simulink model "c_slow_test_cases"  (R2017a)
settings: Solver=FixedStepDiscrete  StartTime=0  StopTime=1000/5e6  RelTol=1e-3
libraries: helperLib x2, simulink x2, commrandsrc3 x2, dspsrcs4 x2
settings Model: FPTRunName=FPA_Reference  SimulationMode=accelerator  ExtModeTrigDuration=100  Creator=cyarp  LastModifiedBy=cyarp
settings SolverCC: InsertRTBMode=Always
settings DataIOCC: LimitDataPoints=on  SaveFinalState=on  SaveFormat=StructureWithTime  SaveOutput=off  SaveState=on  StateSaveName=tmp_raccel_xout  SignalLoggingName=tmp_raccel_logsout
settings OptimizationCC: BlockReduction=off  ConditionallyExecuteInputs=off  DefaultParameterBehavior=Inlined  EfficientMapNaN2IntZero=off  LifeSpan=inf  SimCompilerOptimization=on
settings DebuggingCC: AlgebraicLoopMsg=error  SolverPrmCheckMsg=warning  SingleTaskRateTransMsg=error  SFUnexpectedBacktrackingDiag=warning  SFNoUnconditionalDefaultTransitionDiag=warning  SFExecutionAtInitializationDiag=none
settings HardwareCC: ProdBitPerPointer=32  ProdBitPerSizeT=32  ProdBitPerPtrDiffT=32  ProdLargestAtomicFloat=None  ProdIntDivRoundTo=Undefined  ProdEndianess=Unspecified  ProdWordSize=32  ProdHWDeviceType=ASIC/FPGA->ASIC/FPGA  TargetBitPerPointer=64  TargetBitPerSizeT=64  TargetBitPerPtrDiffT=64  TargetLongLongMode=on  TargetIntDivRoundTo=Zero  TargetEndianess=LittleEndian  TargetWordSize=64  TargetHWDeviceType=MATLAB Host  ProdEqTarget=off
settings ModelReferenceCC: PropagateSignalLabelsOutOfModel=off
settings RTWCC: SystemTargetFile=raccel.tlc  TemplateMakefile=raccel_default_tmf  RTWVerbose=off  RTWUseSimCustomCode=on
settings CodeAppCC: GenerateComments=off  MaxIdLength=128  SimulinkBlockComments=off
settings RaccelTargetCC: GeneratePreprocessorConditionals=Use local settings  ERTFirstTimeCompliant=off  MultiInstanceERTCode=off  ExtModeMexArgs='', 0, 55180  ENABLE_SLEXEC_SSBRIDGE=11  RTWCAPISignals=off  RTWCAPIParams=on
settings ConfigComp: CovMetricSettings=dw  CovHtmlReporting=on  CovSaveCumulativeToWorkspaceVar=on  CovSaveSingleToWorkspaceVar=on  CovExternalEMLEnable=off  CovSFcnEnable=off

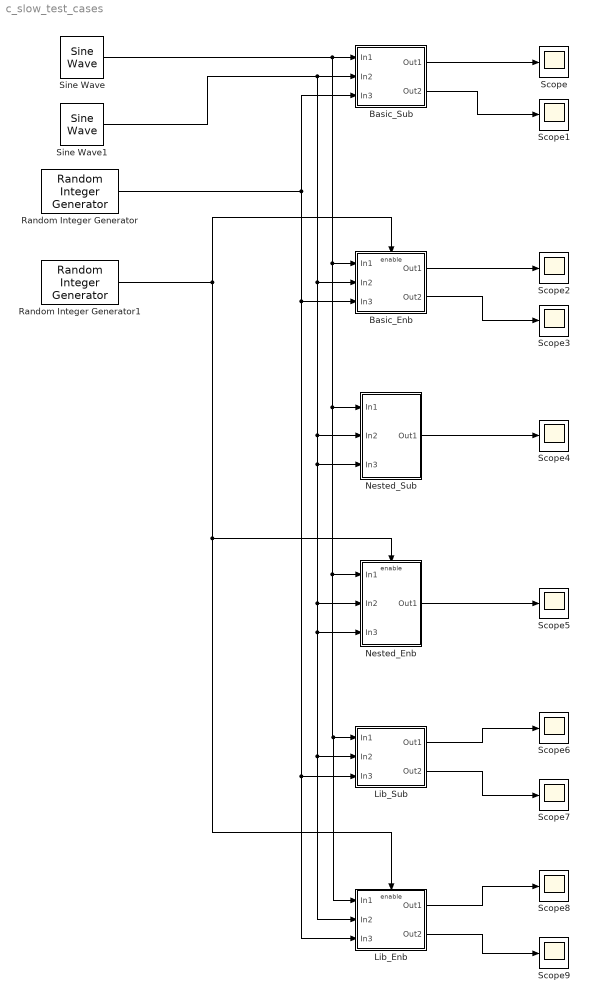
== system c_slow_test_cases ==
  Basic_Enb : Subsystem
  Basic_Sub : Subsystem
  Lib_Enb : Subsystem
  Lib_Sub : Subsystem
  Nested_Enb : Subsystem
  Nested_Sub : Subsystem
  Random Integer Generator : commrandsrc3/Random Integer Generator  SetSize=2  SeedSource=Auto  Seed=0  SampleTime=1/5e6  SamplesPerFrame=1  OutputDataType=boolean  SimulateUsing=Interpreted execution
  Random Integer Generator1 : commrandsrc3/Random Integer Generator  SetSize=2  SeedSource=Auto  Seed=0  SampleTime=1/5e6  SamplesPerFrame=1  OutputDataType=boolean  SimulateUsing=Interpreted execution
  Scope{,1..9} (10 alike) : Scope
  Sine Wave : dspsrcs4/Sine Wave  Amplitude=1  Frequency=10000  Phase=0  SampleMode=Discrete  OutComplex=Complex  CompMethod=Table lookup  TableSize=Speed  SampleTime=1/5e6  SamplesPerFrame=1  ResetState=Restart at time zero  OutputFrames=off  dataType=Fixed-point  wordLen=14  udDataType=sfix(16)  fracBitsMode=User-defined  numFracBits=11  OutDataTypeStr=fixdt(1,14,11)  LastOutDataTypeStr=fixdt(1,14,11)
  Sine Wave1 : dspsrcs4/Sine Wave  Amplitude=1  Frequency=200000  Phase=0  SampleMode=Discrete  OutComplex=Complex  CompMethod=Table lookup  TableSize=Speed  SampleTime=1/5e6  SamplesPerFrame=1  ResetState=Restart at time zero  OutputFrames=off  dataType=Fixed-point  wordLen=14  udDataType=sfix(16)  fracBitsMode=User-defined  numFracBits=11  OutDataTypeStr=fixdt(1,14,11)  LastOutDataTypeStr=fixdt(1,14,11)
  wires:
  Sine Wave/1 -> Nested_Sub/1(In1), Lib_Enb/1(In1), Lib_Sub/1(In1), Nested_Enb/1(In1), Basic_Enb/1(In1), Basic_Sub/1(In1)
  Random Integer Generator/1 -> Lib_Enb/3(In3), Lib_Sub/3(In3), Basic_Enb/3(In3), Basic_Sub/3(In3)
  Basic_Sub/1(Out1) -> Scope/1
  Basic_Sub/2(Out2) -> Scope1/1
  Sine Wave1/1 -> Nested_Sub/2(In2), Nested_Sub/3(In3), Lib_Enb/2(In2), Lib_Sub/2(In2), Nested_Enb/3(In3), Nested_Enb/2(In2), Basic_Enb/2(In2), Basic_Sub/2(In2)
  Random Integer Generator1/1 -> Lib_Enb/Enable, Nested_Enb/Enable, Basic_Enb/Enable
  Basic_Enb/1(Out1) -> Scope2/1
  Basic_Enb/2(Out2) -> Scope3/1
  Nested_Sub/1(Out1) -> Scope4/1
  Nested_Enb/1(Out1) -> Scope5/1
  Lib_Sub/1(Out1) -> Scope6/1
  Lib_Sub/2(Out2) -> Scope7/1
  Lib_Enb/1(Out1) -> Scope8/1
  Lib_Enb/2(Out2) -> Scope9/1

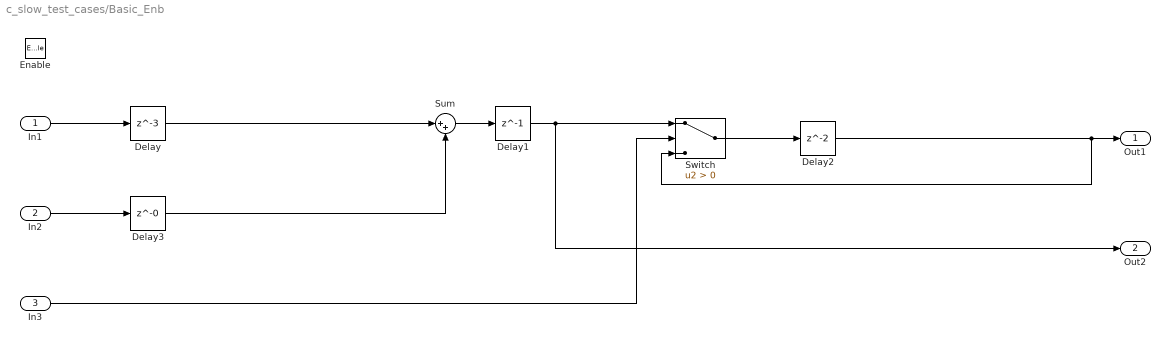
== system c_slow_test_cases/Basic_Enb ==
  In1 : Inport
  In2 : Inport  Port=2
  In3 : Inport  Port=3
  Enable : EnablePort
  Delay : Delay  DelayLength=3  InitialCondition=0
  Delay1 : Delay  DelayLength=1  InitialCondition=0
  Delay2 : Delay  InitialCondition=0
  Delay3 : Delay  DelayLength=0  InitialCondition=0
  Sum : Sum  Inputs=|++  OutDataTypeStr=Inherit: Same as first input
  Switch : Switch  Criteria=u2 > Threshold
  Out1 : Outport
  Out2 : Outport  Port=2
  wires:
  Delay1/1 -> Out2/1, Switch/1
  Switch/1 -> Delay2/1
  Delay2/1 -> Out1/1, Switch/3
  In3/1 -> Switch/2
  Delay/1 -> Sum/1
  In2/1 -> Delay3/1
  In1/1 -> Delay/1
  Sum/1 -> Delay1/1
  Delay3/1 -> Sum/2

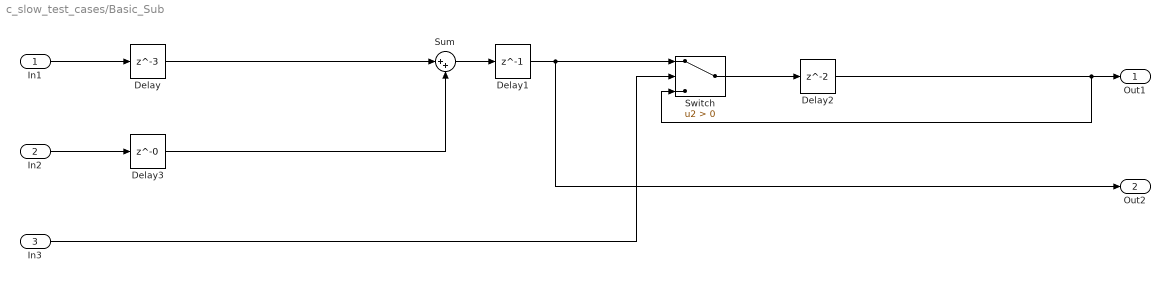
== system c_slow_test_cases/Basic_Sub ==
  In1 : Inport
  In2 : Inport  Port=2
  In3 : Inport  Port=3
  Delay : Delay  DelayLength=3  InitialCondition=0
  Delay1 : Delay  DelayLength=1  InitialCondition=0
  Delay2 : Delay  InitialCondition=0
  Delay3 : Delay  DelayLength=0  InitialCondition=0
  Sum : Sum  Inputs=|++  OutDataTypeStr=Inherit: Same as first input
  Switch : Switch  Criteria=u2 > Threshold
  Out1 : Outport
  Out2 : Outport  Port=2
  wires:
  Delay1/1 -> Out2/1, Switch/1
  Switch/1 -> Delay2/1
  Delay2/1 -> Out1/1, Switch/3
  In3/1 -> Switch/2
  Delay/1 -> Sum/1
  In2/1 -> Delay3/1
  In1/1 -> Delay/1
  Sum/1 -> Delay1/1
  Delay3/1 -> Sum/2

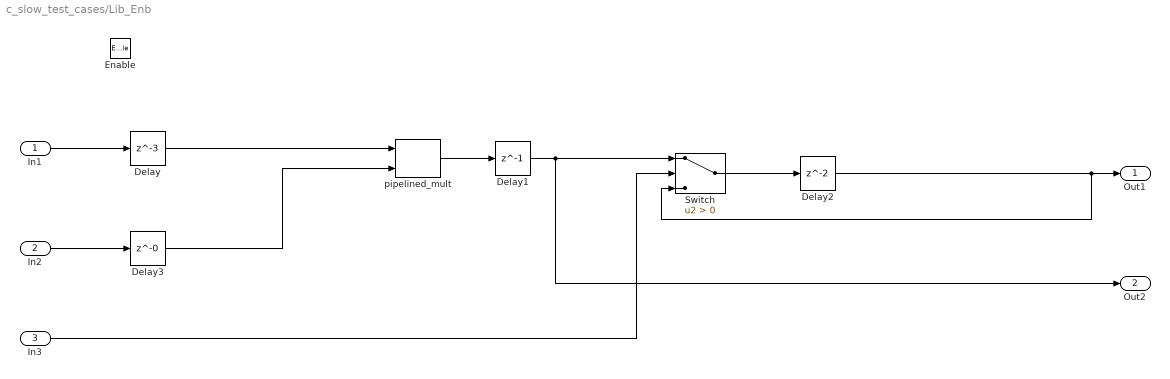
== system c_slow_test_cases/Lib_Enb ==
  In1 : Inport
  In2 : Inport  Port=2
  In3 : Inport  Port=3
  Enable : EnablePort
  Delay : Delay  DelayLength=3  InitialCondition=0
  Delay1 : Delay  DelayLength=1  InitialCondition=0
  Delay2 : Delay  InitialCondition=0
  Delay3 : Delay  DelayLength=0  InitialCondition=0
  Switch : Switch  Criteria=u2 > Threshold
  pipelined_mult : helperLib/pipelined_mult  d=3
  Out1 : Outport
  Out2 : Outport  Port=2
  wires:
  Delay1/1 -> Out2/1, Switch/1
  Switch/1 -> Delay2/1
  Delay2/1 -> Out1/1, Switch/3
  In3/1 -> Switch/2
  In2/1 -> Delay3/1
  In1/1 -> Delay/1
  pipelined_mult/1 -> Delay1/1
  Delay/1 -> pipelined_mult/1
  Delay3/1 -> pipelined_mult/2

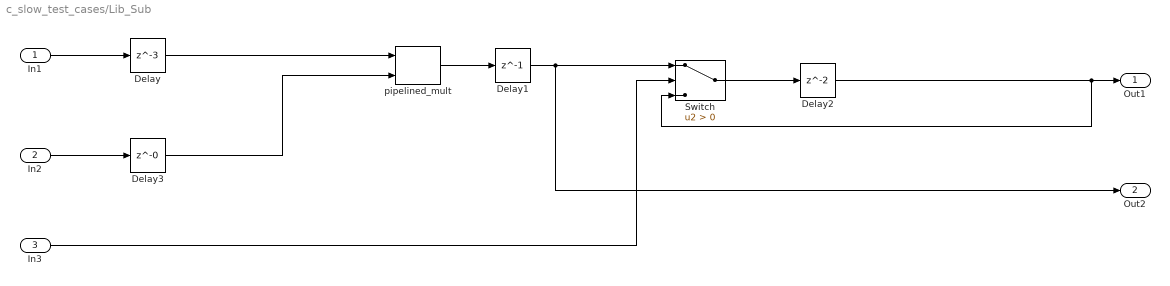
== system c_slow_test_cases/Lib_Sub ==
  In1 : Inport
  In2 : Inport  Port=2
  In3 : Inport  Port=3
  Delay : Delay  DelayLength=3  InitialCondition=0
  Delay1 : Delay  DelayLength=1  InitialCondition=0
  Delay2 : Delay  InitialCondition=0
  Delay3 : Delay  DelayLength=0  InitialCondition=0
  Switch : Switch  Criteria=u2 > Threshold
  pipelined_mult : helperLib/pipelined_mult  d=3
  Out1 : Outport
  Out2 : Outport  Port=2
  wires:
  Delay1/1 -> Out2/1, Switch/1
  Switch/1 -> Delay2/1
  Delay2/1 -> Out1/1, Switch/3
  In3/1 -> Switch/2
  In2/1 -> Delay3/1
  In1/1 -> Delay/1
  pipelined_mult/1 -> Delay1/1
  Delay/1 -> pipelined_mult/1
  Delay3/1 -> pipelined_mult/2

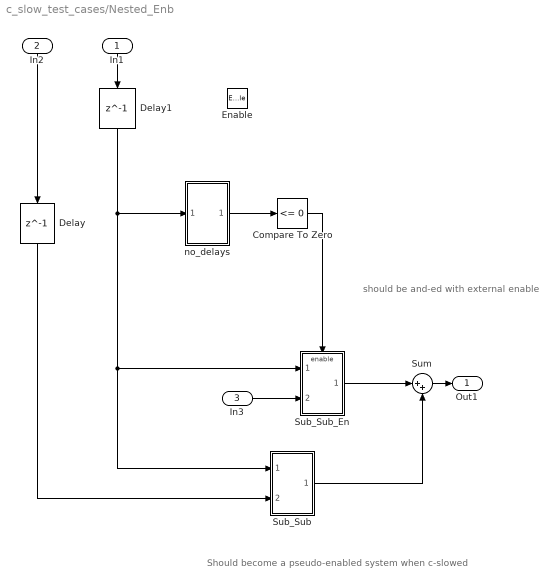
== system c_slow_test_cases/Nested_Enb ==
  note: should be and-ed with external enable
  note: Should become a pseudo-enabled system when c-slowed
  In1 : Inport
  In2 : Inport  Port=2
  In3 : Inport  Port=3
  Enable : EnablePort
  Compare To Zero : simulink/Logic and Bit Operations/Compare To Zero  relop=<=  OutDataTypeStr=boolean
  Delay : Delay  DelayLength=1  InitialCondition=0
  Delay1 : Delay  DelayLength=1  InitialCondition=0
  Sub_Sub : Subsystem
  Sub_Sub_En : Subsystem
  Sum : Sum  Inputs=|++  OutDataTypeStr=Inherit: Same as first input
  no_delays : Subsystem
  Out1 : Outport
  wires:
  Sum/1 -> Out1/1
  Sub_Sub/1(Out1) -> Sum/2
  Sub_Sub_En/1(Out1) -> Sum/1
  Compare To Zero/1 -> Sub_Sub_En/Enable
  In3/1 -> Sub_Sub_En/2(In2)
  no_delays/1(Out1) -> Compare To Zero/1
  Delay/1 -> Sub_Sub/2(In2)
  Delay1/1 -> no_delays/1(In1), Sub_Sub_En/1(In1), Sub_Sub/1(In1)
  In2/1 -> Delay/1
  In1/1 -> Delay1/1

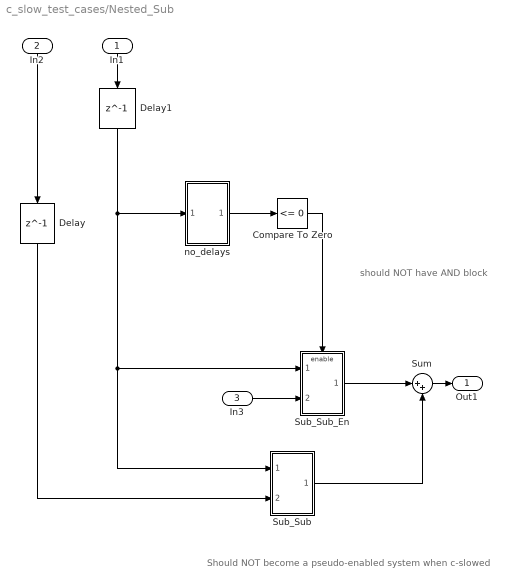
== system c_slow_test_cases/Nested_Sub ==
  note: should NOT have AND block
  note: Should NOT become a pseudo-enabled system when c-slowed
  In1 : Inport
  In2 : Inport  Port=2
  In3 : Inport  Port=3
  Compare To Zero : simulink/Logic and Bit Operations/Compare To Zero  relop=<=  OutDataTypeStr=boolean
  Delay : Delay  DelayLength=1  InitialCondition=0
  Delay1 : Delay  DelayLength=1  InitialCondition=0
  Sub_Sub : Subsystem
  Sub_Sub_En : Subsystem
  Sum : Sum  Inputs=|++  OutDataTypeStr=Inherit: Same as first input
  no_delays : Subsystem
  Out1 : Outport
  wires:
  Sum/1 -> Out1/1
  Sub_Sub/1(Out1) -> Sum/2
  Sub_Sub_En/1(Out1) -> Sum/1
  Compare To Zero/1 -> Sub_Sub_En/Enable
  In3/1 -> Sub_Sub_En/2(In2)
  no_delays/1(Out1) -> Compare To Zero/1
  Delay/1 -> Sub_Sub/2(In2)
  Delay1/1 -> no_delays/1(In1), Sub_Sub_En/1(In1), Sub_Sub/1(In1)
  In2/1 -> Delay/1
  In1/1 -> Delay1/1

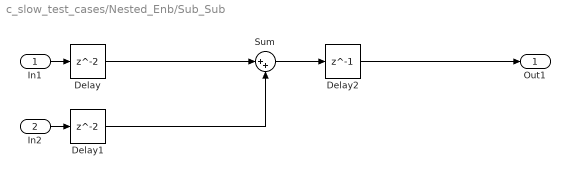
== system c_slow_test_cases/Nested_Enb/Sub_Sub ==
  In1 : Inport
  In2 : Inport  Port=2
  Delay : Delay  InitialCondition=0
  Delay1 : Delay  InitialCondition=0
  Delay2 : Delay  DelayLength=1  InitialCondition=0
  Sum : Sum  Inputs=|++  OutDataTypeStr=Inherit: Same as first input
  Out1 : Outport
  wires:
  Delay/1 -> Sum/1
  In2/1 -> Delay1/1
  Delay2/1 -> Out1/1
  Sum/1 -> Delay2/1
  Delay1/1 -> Sum/2
  In1/1 -> Delay/1

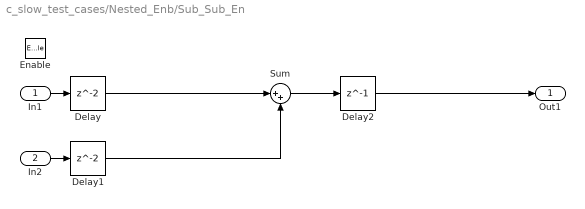
== system c_slow_test_cases/Nested_Enb/Sub_Sub_En ==
  In1 : Inport
  In2 : Inport  Port=2
  Enable : EnablePort
  Delay : Delay  InitialCondition=0
  Delay1 : Delay  InitialCondition=0
  Delay2 : Delay  DelayLength=1  InitialCondition=0
  Sum : Sum  Inputs=|++  OutDataTypeStr=Inherit: Same as first input
  Out1 : Outport
  wires:
  Delay/1 -> Sum/1
  In2/1 -> Delay1/1
  Delay2/1 -> Out1/1
  Sum/1 -> Delay2/1
  Delay1/1 -> Sum/2
  In1/1 -> Delay/1

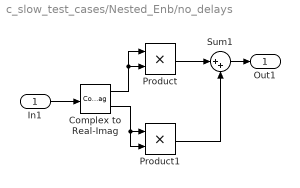
== system c_slow_test_cases/Nested_Enb/no_delays ==
  In1 : Inport
  Complex to Real-Imag : ComplexToRealImag
  Product : Product
  Product1 : Product
  Sum1 : Sum  Inputs=|++  OutDataTypeStr=Inherit: Same as first input
  Out1 : Outport
  wires:
  Complex to Real-Imag/2 -> Product1/2, Product1/1
  Product1/1 -> Sum1/2
  Sum1/1 -> Out1/1
  Complex to Real-Imag/1 -> Product/1, Product/2
  In1/1 -> Complex to Real-Imag/1
  Product/1 -> Sum1/1

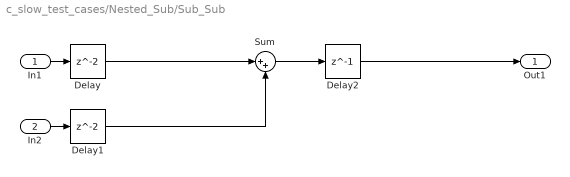
== system c_slow_test_cases/Nested_Sub/Sub_Sub ==
  In1 : Inport
  In2 : Inport  Port=2
  Delay : Delay  InitialCondition=0
  Delay1 : Delay  InitialCondition=0
  Delay2 : Delay  DelayLength=1  InitialCondition=0
  Sum : Sum  Inputs=|++  OutDataTypeStr=Inherit: Same as first input
  Out1 : Outport
  wires:
  Delay/1 -> Sum/1
  In2/1 -> Delay1/1
  Delay2/1 -> Out1/1
  Sum/1 -> Delay2/1
  Delay1/1 -> Sum/2
  In1/1 -> Delay/1

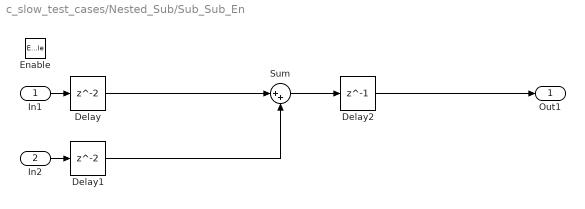
== system c_slow_test_cases/Nested_Sub/Sub_Sub_En ==
  In1 : Inport
  In2 : Inport  Port=2
  Enable : EnablePort
  Delay : Delay  InitialCondition=0
  Delay1 : Delay  InitialCondition=0
  Delay2 : Delay  DelayLength=1  InitialCondition=0
  Sum : Sum  Inputs=|++  OutDataTypeStr=Inherit: Same as first input
  Out1 : Outport
  wires:
  Delay/1 -> Sum/1
  In2/1 -> Delay1/1
  Delay2/1 -> Out1/1
  Sum/1 -> Delay2/1
  Delay1/1 -> Sum/2
  In1/1 -> Delay/1

== system c_slow_test_cases/Nested_Sub/no_delays ==
  In1 : Inport
  Complex to Real-Imag : ComplexToRealImag
  Product : Product
  Product1 : Product
  Sum1 : Sum  Inputs=|++  OutDataTypeStr=Inherit: Same as first input
  Out1 : Outport
  wires:
  Complex to Real-Imag/2 -> Product1/2, Product1/1
  Product1/1 -> Sum1/2
  Sum1/1 -> Out1/1
  Complex to Real-Imag/1 -> Product/1, Product/2
  In1/1 -> Complex to Real-Imag/1
  Product/1 -> Sum1/1
